simulink model "test"  (R2023a)
settings: Solver=FixedStepDiscrete  StartTime=0.0  StopTime=10.0  FixedStep=.1  RelTol=1e-3
model workspace (MAT data in the model file):
  delayedLen = 10
settings Model: Creator=92371  LastModifiedBy=92371

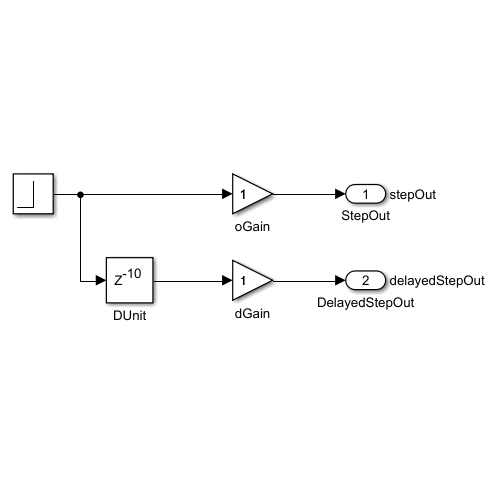
[thumbnail: Simulink's stored preview of the top-level diagram]
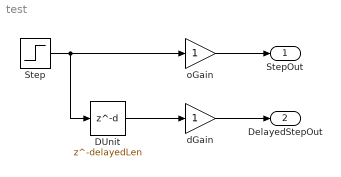
== system test ==
  DUnit : Delay  DelayLength=delayedLen
  Step : Step  SampleTime=0
  dGain : Gain
  oGain : Gain
  StepOut : Outport  SignalName=stepOut
  DelayedStepOut : Outport  Port=2  SignalName=delayedStepOut
  wires:
  Step/1 -> oGain/1, DUnit/1
  DUnit/1 -> dGain/1
  oGain/1 -> StepOut/1
  dGain/1 -> DelayedStepOut/1
